simulink model "prob3"  (R2020b)
settings: Solver=VariableStepAuto  StartTime=0.0  StopTime=10.0  RelTol=1e-3
libraries: simulink x1
settings Model: Creator=parke  LastModifiedBy=parke

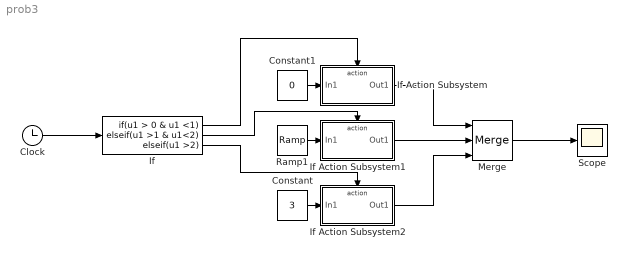
== system prob3 ==
  Clock : Clock
  Constant : Constant  Value=3
  Constant1 : Constant  Value=0
  If : If  IfExpression=u1 > 0 & u1 <1  ElseIfExpressions=u1 >1 & u1<2 , u1 >2  ShowElse=off
  If Action Subsystem : Subsystem  TreatAsAtomicUnit=on
  If Action Subsystem1 : Subsystem  TreatAsAtomicUnit=on
  If Action Subsystem2 : Subsystem  TreatAsAtomicUnit=on
  Merge : Merge  Inputs=3
  Ramp1 : simulink/Sources/Ramp  slope=3  start=1  InitialOutput=0
  Scope : Scope
  wires:
  Clock/1 -> If/1
  Constant/1 -> If Action Subsystem2/1(In1)
  If Action Subsystem1/1(Out1) -> Merge/2
  If/2 -> If Action Subsystem1/Action
  If Action Subsystem2/1(Out1) -> Merge/3
  If Action Subsystem/1(Out1) -> Merge/1
  If/3 -> If Action Subsystem2/Action
  Ramp1/1 -> If Action Subsystem1/1(In1)
  If/1 -> If Action Subsystem/Action
  Constant1/1 -> If Action Subsystem/1(In1)
  Merge/1 -> Scope/1

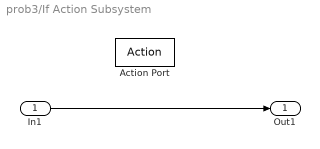
== system prob3/If Action Subsystem ==
  In1 : Inport
  Action Port : ActionPort  ActionPortLabel=if(u1 > 0 & u1 <1)
  Out1 : Outport
  wires:
  In1/1 -> Out1/1

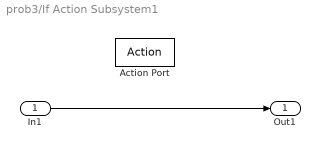
== system prob3/If Action Subsystem1 ==
  In1 : Inport
  Action Port : ActionPort  ActionPortLabel=elseif(u1 >1 & u1<2 )
  Out1 : Outport
  wires:
  In1/1 -> Out1/1

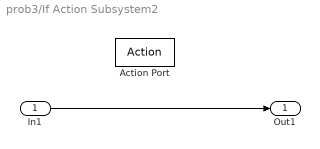
== system prob3/If Action Subsystem2 ==
  In1 : Inport
  Action Port : ActionPort  ActionPortLabel="elseif( u1 >2  )"
  Out1 : Outport
  wires:
  In1/1 -> Out1/1
